simulink library "rov_design_analysis"  (Simulink 6.0)
settings: Solver=ode45  SolverMode=SingleTasking  StartTime=0.0  StopTime=10.0  RelTol=1e-3
undefined symbols (not defined in the file or in its folder): amp, At, B, Bt, Ct, cycles, D, den, DL, Do, DQ, DQL, freq, frtest, I, L, m, M, Ma, magnitude, MaU, Mt, nmiss, num, phase, rg, sigbuilder_block, slcm, T, W, xb, xg, Xudot, yb, yg, Yvdot, zb, zg, Zwdot
libraries: simulink_extras x32, simulink x27, rov_design_analysis x15, marine_gnc x10, dspmtrx2 x6, dspstat3 x4
(part 6 of 9)

== system rov_design_analysis/ROV Controller /Hybrid Control- one DoF/Body-fixed to Earth_fixed Transformation1/Transformation matrix T ==
  translational body velocity : Inport  Port=1  LatchInput=off
  angular position : Inport  Port=2  LatchInput=off
  Mux : Mux  Inputs=3
  Row1 of R : Subsystem
      mask Display: disp('Row 1')
  Row2 of R : Subsystem
      mask Display: disp('Row 2')
  Row3 of R : Subsystem
      mask Display: disp('Row 3')
  translational earth velocity : Outport  InitialOutput=0
  wires:
  Mux/1 -> translational earth velocity/1
  Row3 of R/1(translational earth velocity (row 3)) -> Mux/3
  Row2 of R/1(translational earth velocity (row 2)) -> Mux/2
  Row1 of R/1(translational earth velocity (row 1)) -> Mux/1
  angular position/1 -> Row3 of R/2(angular position), Row1 of R/2(angular position), Row2 of R/2(angular position)
  translational body velocity/1 -> Row1 of R/1(translational body velocity), Row2 of R/1(translational body velocity), Row3 of R/1(translational body velocity)

== system rov_design_analysis/ROV Controller /Hybrid Control- one DoF/Body-fixed to Earth_fixed Transformation3/Transformation matrix R ==
  angular body  velocity : Inport  Port=1  LatchInput=off
  angular position : Inport  Port=2  LatchInput=off
  Mux : Mux  Inputs=3
  Row1 of T : Subsystem
      mask Display: disp('Row 1')
  Row2 of T : Subsystem
      mask Display: disp('Row 2')
  Row3 of T : Subsystem
      mask Display: disp('Row 3')
  angular earth velocity : Outport  InitialOutput=0
  wires:
  angular body  velocity/1 -> Row1 of T/1(angular body  velocity), Row2 of T/1("angular body velocity "), Row3 of T/1("angular body velocity ")
  Row1 of T/1(angular earth velocity (row 1)) -> Mux/1
  Row2 of T/1(angular earth velocity (row 2)) -> Mux/2
  Row3 of T/1(angular earth velocity (row 3)) -> Mux/3
  Mux/1 -> angular earth velocity/1
  angular position/1 -> Row2 of T/2(angular position), Row1 of T/2(angular position), Row3 of T/2(angular position)

== system rov_design_analysis/ROV Controller /Hybrid Control- one DoF/Body-fixed to Earth_fixed Transformation3/Transformation matrix T ==
  translational body velocity : Inport  Port=1  LatchInput=off
  angular position : Inport  Port=2  LatchInput=off
  Mux : Mux  Inputs=3
  Row1 of R : Subsystem
      mask Display: disp('Row 1')
  Row2 of R : Subsystem
      mask Display: disp('Row 2')
  Row3 of R : Subsystem
      mask Display: disp('Row 3')
  translational earth velocity : Outport  InitialOutput=0
  wires:
  translational body velocity/1 -> Row3 of R/1(translational body velocity), Row2 of R/1(translational body velocity), Row1 of R/1(translational body velocity)
  angular position/1 -> Row2 of R/2(angular position), Row1 of R/2(angular position), Row3 of R/2(angular position)
  Row1 of R/1(translational earth velocity (row 1)) -> Mux/1
  Row2 of R/1(translational earth velocity (row 2)) -> Mux/2
  Row3 of R/1(translational earth velocity (row 3)) -> Mux/3
  Mux/1 -> translational earth velocity/1

== system rov_design_analysis/ROV Controller /Hybrid Control- one DoF/Subsystem2/SubSystem11 ==
  volt : Inport  Port=1  LatchInput=off
  Transfer Fcn : TransferFcn  Numerator=[3700 0.037]  Denominator=[0.5 847.5 76000]
  thrust : Outport
  wires:
  Transfer Fcn/1 -> thrust/1
  volt/1 -> Transfer Fcn/1

== system rov_design_analysis/ROV Controller /Hybrid Control- one DoF/Subsystem2/SubSystem12 ==
  volt : Inport  Port=1  LatchInput=off
  Transfer Fcn : TransferFcn  Numerator=[3700 0.037]  Denominator=[0.5 847.5 76000]
  thrust : Outport
  wires:
  Transfer Fcn/1 -> thrust/1
  volt/1 -> Transfer Fcn/1

== system rov_design_analysis/ROV Controller /Hybrid Control- one DoF/Subsystem2/SubSystem5 ==
  volt : Inport  Port=1  LatchInput=off
  Transfer Fcn : TransferFcn  Numerator=[3700 0.037]  Denominator=[0.5 847.5 76000]
  thrust : Outport
  wires:
  Transfer Fcn/1 -> thrust/1
  volt/1 -> Transfer Fcn/1

== system rov_design_analysis/ROV Controller /Hybrid Control- one DoF/Subsystem2/SubSystem6 ==
  volt : Inport  Port=1  LatchInput=off
  Transfer Fcn : TransferFcn  Numerator=[3700 0.037]  Denominator=[0.5 847.5 76000]
  thrust : Outport
  wires:
  Transfer Fcn/1 -> thrust/1
  volt/1 -> Transfer Fcn/1

== system rov_design_analysis/ROV Controller /Nonlinear-Based PD  Cascaded  Controller - 6 DoF/Body-fixed to Earth_fixed Transformation1/Transformation matrix R ==
  angular body  velocity : Inport  Port=1  LatchInput=off
  angular position : Inport  Port=2  LatchInput=off
  Mux : Mux  Inputs=3
  Row1 of T : Subsystem
      mask Display: disp('Row 1')
  Row2 of T : Subsystem
      mask Display: disp('Row 2')
  Row3 of T : Subsystem
      mask Display: disp('Row 3')
  angular earth velocity : Outport  InitialOutput=0
  wires:
  angular position/1 -> Row3 of T/2(angular position), Row1 of T/2(angular position), Row2 of T/2(angular position)
  Mux/1 -> angular earth velocity/1
  Row3 of T/1(angular earth velocity (row 3)) -> Mux/3
  Row2 of T/1(angular earth velocity (row 2)) -> Mux/2
  Row1 of T/1(angular earth velocity (row 1)) -> Mux/1
  angular body  velocity/1 -> Row3 of T/1("angular body velocity "), Row2 of T/1("angular body velocity "), Row1 of T/1(angular body  velocity)

== system rov_design_analysis/ROV Controller /Nonlinear-Based PD  Cascaded  Controller - 6 DoF/Body-fixed to Earth_fixed Transformation1/Transformation matrix T ==
  translational body velocity : Inport  Port=1  LatchInput=off
  angular position : Inport  Port=2  LatchInput=off
  Mux : Mux  Inputs=3
  Row1 of R : Subsystem
      mask Display: disp('Row 1')
  Row2 of R : Subsystem
      mask Display: disp('Row 2')
  Row3 of R : Subsystem
      mask Display: disp('Row 3')
  translational earth velocity : Outport  InitialOutput=0
  wires:
  Mux/1 -> translational earth velocity/1
  Row3 of R/1(translational earth velocity (row 3)) -> Mux/3
  Row2 of R/1(translational earth velocity (row 2)) -> Mux/2
  Row1 of R/1(translational earth velocity (row 1)) -> Mux/1
  angular position/1 -> Row3 of R/2(angular position), Row1 of R/2(angular position), Row2 of R/2(angular position)
  translational body velocity/1 -> Row1 of R/1(translational body velocity), Row2 of R/1(translational body velocity), Row3 of R/1(translational body velocity)

== system rov_design_analysis/ROV Controller /Nonlinear-Based PD  Cascaded  Controller - 6 DoF/Body-fixed to Earth_fixed Transformation3/Transformation matrix R ==
  angular body  velocity : Inport  Port=1  LatchInput=off
  angular position : Inport  Port=2  LatchInput=off
  Mux : Mux  Inputs=3
  Row1 of T : Subsystem
      mask Display: disp('Row 1')
  Row2 of T : Subsystem
      mask Display: disp('Row 2')
  Row3 of T : Subsystem
      mask Display: disp('Row 3')
  angular earth velocity : Outport  InitialOutput=0
  wires:
  angular body  velocity/1 -> Row1 of T/1(angular body  velocity), Row2 of T/1("angular body velocity "), Row3 of T/1("angular body velocity ")
  Row1 of T/1(angular earth velocity (row 1)) -> Mux/1
  Row2 of T/1(angular earth velocity (row 2)) -> Mux/2
  Row3 of T/1(angular earth velocity (row 3)) -> Mux/3
  Mux/1 -> angular earth velocity/1
  angular position/1 -> Row2 of T/2(angular position), Row1 of T/2(angular position), Row3 of T/2(angular position)

== system rov_design_analysis/ROV Controller /Nonlinear-Based PD  Cascaded  Controller - 6 DoF/Body-fixed to Earth_fixed Transformation3/Transformation matrix T ==
  translational body velocity : Inport  Port=1  LatchInput=off
  angular position : Inport  Port=2  LatchInput=off
  Mux : Mux  Inputs=3
  Row1 of R : Subsystem
      mask Display: disp('Row 1')
  Row2 of R : Subsystem
      mask Display: disp('Row 2')
  Row3 of R : Subsystem
      mask Display: disp('Row 3')
  translational earth velocity : Outport  InitialOutput=0
  wires:
  translational body velocity/1 -> Row3 of R/1(translational body velocity), Row2 of R/1(translational body velocity), Row1 of R/1(translational body velocity)
  angular position/1 -> Row2 of R/2(angular position), Row1 of R/2(angular position), Row3 of R/2(angular position)
  Row1 of R/1(translational earth velocity (row 1)) -> Mux/1
  Row2 of R/1(translational earth velocity (row 2)) -> Mux/2
  Row3 of R/1(translational earth velocity (row 3)) -> Mux/3
  Mux/1 -> translational earth velocity/1

== system rov_design_analysis/ROV Controller /Nonlinear-Based PD  Cascaded  Controller - 6 DoF/Subsystem2/SubSystem11 ==
  volt : Inport  Port=1  LatchInput=off
  Transfer Fcn : TransferFcn  Numerator=[3700 0.037]  Denominator=[0.5 847.5 76000]
  thrust : Outport
  wires:
  Transfer Fcn/1 -> thrust/1
  volt/1 -> Transfer Fcn/1

== system rov_design_analysis/ROV Controller /Nonlinear-Based PD  Cascaded  Controller - 6 DoF/Subsystem2/SubSystem12 ==
  volt : Inport  Port=1  LatchInput=off
  Transfer Fcn : TransferFcn  Numerator=[3700 0.037]  Denominator=[0.5 847.5 76000]
  thrust : Outport
  wires:
  Transfer Fcn/1 -> thrust/1
  volt/1 -> Transfer Fcn/1

== system rov_design_analysis/ROV Controller /Nonlinear-Based PD  Cascaded  Controller - 6 DoF/Subsystem2/SubSystem5 ==
  volt : Inport  Port=1  LatchInput=off
  Transfer Fcn : TransferFcn  Numerator=[3700 0.037]  Denominator=[0.5 847.5 76000]
  thrust : Outport
  wires:
  Transfer Fcn/1 -> thrust/1
  volt/1 -> Transfer Fcn/1

== system rov_design_analysis/ROV Controller /Nonlinear-Based PD  Cascaded  Controller - 6 DoF/Subsystem2/SubSystem6 ==
  volt : Inport  Port=1  LatchInput=off
  Transfer Fcn : TransferFcn  Numerator=[3700 0.037]  Denominator=[0.5 847.5 76000]
  thrust : Outport
  wires:
  Transfer Fcn/1 -> thrust/1
  volt/1 -> Transfer Fcn/1

== system rov_design_analysis/ROV Controller /Nonlinear-Sliding-Mode Cascaded  Controller - 6 DoF/Body-fixed to Earth_fixed Transformation1/Transformation matrix R ==
  angular body  velocity : Inport  Port=1  LatchInput=off
  angular position : Inport  Port=2  LatchInput=off
  Mux : Mux  Inputs=3
  Row1 of T : Subsystem
      mask Display: disp('Row 1')
  Row2 of T : Subsystem
      mask Display: disp('Row 2')
  Row3 of T : Subsystem
      mask Display: disp('Row 3')
  angular earth velocity : Outport  InitialOutput=0
  wires:
  angular body  velocity/1 -> Row1 of T/1(angular body  velocity), Row2 of T/1("angular body velocity "), Row3 of T/1("angular body velocity ")
  Row1 of T/1(angular earth velocity (row 1)) -> Mux/1
  Row2 of T/1(angular earth velocity (row 2)) -> Mux/2
  Row3 of T/1(angular earth velocity (row 3)) -> Mux/3
  Mux/1 -> angular earth velocity/1
  angular position/1 -> Row2 of T/2(angular position), Row1 of T/2(angular position), Row3 of T/2(angular position)

== system rov_design_analysis/ROV Controller /Nonlinear-Sliding-Mode Cascaded  Controller - 6 DoF/Body-fixed to Earth_fixed Transformation1/Transformation matrix T ==
  translational body velocity : Inport  Port=1  LatchInput=off
  angular position : Inport  Port=2  LatchInput=off
  Mux : Mux  Inputs=3
  Row1 of R : Subsystem
      mask Display: disp('Row 1')
  Row2 of R : Subsystem
      mask Display: disp('Row 2')
  Row3 of R : Subsystem
      mask Display: disp('Row 3')
  translational earth velocity : Outport  InitialOutput=0
  wires:
  translational body velocity/1 -> Row3 of R/1(translational body velocity), Row2 of R/1(translational body velocity), Row1 of R/1(translational body velocity)
  angular position/1 -> Row2 of R/2(angular position), Row1 of R/2(angular position), Row3 of R/2(angular position)
  Row1 of R/1(translational earth velocity (row 1)) -> Mux/1
  Row2 of R/1(translational earth velocity (row 2)) -> Mux/2
  Row3 of R/1(translational earth velocity (row 3)) -> Mux/3
  Mux/1 -> translational earth velocity/1

== system rov_design_analysis/ROV Controller /Nonlinear-Sliding-Mode Cascaded  Controller - 6 DoF/Body-fixed to Earth_fixed Transformation3/Transformation matrix R ==
  angular body  velocity : Inport  Port=1  LatchInput=off
  angular position : Inport  Port=2  LatchInput=off
  Mux : Mux  Inputs=3
  Row1 of T : Subsystem
      mask Display: disp('Row 1')
  Row2 of T : Subsystem
      mask Display: disp('Row 2')
  Row3 of T : Subsystem
      mask Display: disp('Row 3')
  angular earth velocity : Outport  InitialOutput=0
  wires:
  angular position/1 -> Row3 of T/2(angular position), Row1 of T/2(angular position), Row2 of T/2(angular position)
  Mux/1 -> angular earth velocity/1
  Row3 of T/1(angular earth velocity (row 3)) -> Mux/3
  Row2 of T/1(angular earth velocity (row 2)) -> Mux/2
  Row1 of T/1(angular earth velocity (row 1)) -> Mux/1
  angular body  velocity/1 -> Row3 of T/1("angular body velocity "), Row2 of T/1("angular body velocity "), Row1 of T/1(angular body  velocity)

== system rov_design_analysis/ROV Controller /Nonlinear-Sliding-Mode Cascaded  Controller - 6 DoF/Body-fixed to Earth_fixed Transformation3/Transformation matrix T ==
  translational body velocity : Inport  Port=1  LatchInput=off
  angular position : Inport  Port=2  LatchInput=off
  Mux : Mux  Inputs=3
  Row1 of R : Subsystem
      mask Display: disp('Row 1')
  Row2 of R : Subsystem
      mask Display: disp('Row 2')
  Row3 of R : Subsystem
      mask Display: disp('Row 3')
  translational earth velocity : Outport  InitialOutput=0
  wires:
  Mux/1 -> translational earth velocity/1
  Row3 of R/1(translational earth velocity (row 3)) -> Mux/3
  Row2 of R/1(translational earth velocity (row 2)) -> Mux/2
  Row1 of R/1(translational earth velocity (row 1)) -> Mux/1
  angular position/1 -> Row3 of R/2(angular position), Row1 of R/2(angular position), Row2 of R/2(angular position)
  translational body velocity/1 -> Row1 of R/1(translational body velocity), Row2 of R/1(translational body velocity), Row3 of R/1(translational body velocity)

== system rov_design_analysis/ROV Controller /Nonlinear-Sliding-Mode Cascaded  Controller - 6 DoF/Subsystem2/SubSystem11 ==
  volt : Inport  Port=1  LatchInput=off
  Transfer Fcn : TransferFcn  Numerator=[3700 0.037]  Denominator=[0.5 847.5 76000]
  thrust : Outport
  wires:
  volt/1 -> Transfer Fcn/1
  Transfer Fcn/1 -> thrust/1

== system rov_design_analysis/ROV Controller /Nonlinear-Sliding-Mode Cascaded  Controller - 6 DoF/Subsystem2/SubSystem12 ==
  volt : Inport  Port=1  LatchInput=off
  Transfer Fcn : TransferFcn  Numerator=[3700 0.037]  Denominator=[0.5 847.5 76000]
  thrust : Outport
  wires:
  volt/1 -> Transfer Fcn/1
  Transfer Fcn/1 -> thrust/1

== system rov_design_analysis/ROV Controller /Nonlinear-Sliding-Mode Cascaded  Controller - 6 DoF/Subsystem2/SubSystem5 ==
  volt : Inport  Port=1  LatchInput=off
  Transfer Fcn : TransferFcn  Numerator=[3700 0.037]  Denominator=[0.5 847.5 76000]
  thrust : Outport
  wires:
  volt/1 -> Transfer Fcn/1
  Transfer Fcn/1 -> thrust/1

== system rov_design_analysis/ROV Controller /Nonlinear-Sliding-Mode Cascaded  Controller - 6 DoF/Subsystem2/SubSystem6 ==
  volt : Inport  Port=1  LatchInput=off
  Transfer Fcn : TransferFcn  Numerator=[3700 0.037]  Denominator=[0.5 847.5 76000]
  thrust : Outport
  wires:
  volt/1 -> Transfer Fcn/1
  Transfer Fcn/1 -> thrust/1

== system rov_design_analysis/ROV Controller /P-Decoupled  Cascaded loop Controller  - 6 DoF/Body-fixed to Earth_fixed Transformation1/Transformation matrix R ==
  angular body  velocity : Inport  Port=1  LatchInput=off
  angular position : Inport  Port=2  LatchInput=off
  Mux : Mux  Inputs=3
  Row1 of T : Subsystem
      mask Display: disp('Row 1')
  Row2 of T : Subsystem
      mask Display: disp('Row 2')
  Row3 of T : Subsystem
      mask Display: disp('Row 3')
  angular earth velocity : Outport  InitialOutput=0
  wires:
  angular body  velocity/1 -> Row1 of T/1(angular body  velocity), Row2 of T/1("angular body velocity "), Row3 of T/1("angular body velocity ")
  Row1 of T/1(angular earth velocity (row 1)) -> Mux/1
  Row2 of T/1(angular earth velocity (row 2)) -> Mux/2
  Row3 of T/1(angular earth velocity (row 3)) -> Mux/3
  Mux/1 -> angular earth velocity/1
  angular position/1 -> Row2 of T/2(angular position), Row1 of T/2(angular position), Row3 of T/2(angular position)

== system rov_design_analysis/ROV Controller /P-Decoupled  Cascaded loop Controller  - 6 DoF/Body-fixed to Earth_fixed Transformation1/Transformation matrix T ==
  translational body velocity : Inport  Port=1  LatchInput=off
  angular position : Inport  Port=2  LatchInput=off
  Mux : Mux  Inputs=3
  Row1 of R : Subsystem
      mask Display: disp('Row 1')
  Row2 of R : Subsystem
      mask Display: disp('Row 2')
  Row3 of R : Subsystem
      mask Display: disp('Row 3')
  translational earth velocity : Outport  InitialOutput=0
  wires:
  translational body velocity/1 -> Row3 of R/1(translational body velocity), Row2 of R/1(translational body velocity), Row1 of R/1(translational body velocity)
  angular position/1 -> Row2 of R/2(angular position), Row1 of R/2(angular position), Row3 of R/2(angular position)
  Row1 of R/1(translational earth velocity (row 1)) -> Mux/1
  Row2 of R/1(translational earth velocity (row 2)) -> Mux/2
  Row3 of R/1(translational earth velocity (row 3)) -> Mux/3
  Mux/1 -> translational earth velocity/1

== system rov_design_analysis/ROV Controller /P-Decoupled  Cascaded loop Controller  - 6 DoF/Body-fixed to Earth_fixed Transformation3/Transformation matrix R ==
  angular body  velocity : Inport  Port=1  LatchInput=off
  angular position : Inport  Port=2  LatchInput=off
  Mux : Mux  Inputs=3
  Row1 of T : Subsystem
      mask Display: disp('Row 1')
  Row2 of T : Subsystem
      mask Display: disp('Row 2')
  Row3 of T : Subsystem
      mask Display: disp('Row 3')
  angular earth velocity : Outport  InitialOutput=0
  wires:
  angular position/1 -> Row3 of T/2(angular position), Row1 of T/2(angular position), Row2 of T/2(angular position)
  Mux/1 -> angular earth velocity/1
  Row3 of T/1(angular earth velocity (row 3)) -> Mux/3
  Row2 of T/1(angular earth velocity (row 2)) -> Mux/2
  Row1 of T/1(angular earth velocity (row 1)) -> Mux/1
  angular body  velocity/1 -> Row3 of T/1("angular body velocity "), Row2 of T/1("angular body velocity "), Row1 of T/1(angular body  velocity)

== system rov_design_analysis/ROV Controller /P-Decoupled  Cascaded loop Controller  - 6 DoF/Body-fixed to Earth_fixed Transformation3/Transformation matrix T ==
  translational body velocity : Inport  Port=1  LatchInput=off
  angular position : Inport  Port=2  LatchInput=off
  Mux : Mux  Inputs=3
  Row1 of R : Subsystem
      mask Display: disp('Row 1')
  Row2 of R : Subsystem
      mask Display: disp('Row 2')
  Row3 of R : Subsystem
      mask Display: disp('Row 3')
  translational earth velocity : Outport  InitialOutput=0
  wires:
  Mux/1 -> translational earth velocity/1
  Row3 of R/1(translational earth velocity (row 3)) -> Mux/3
  Row2 of R/1(translational earth velocity (row 2)) -> Mux/2
  Row1 of R/1(translational earth velocity (row 1)) -> Mux/1
  angular position/1 -> Row3 of R/2(angular position), Row1 of R/2(angular position), Row2 of R/2(angular position)
  translational body velocity/1 -> Row1 of R/1(translational body velocity), Row2 of R/1(translational body velocity), Row3 of R/1(translational body velocity)

== system rov_design_analysis/ROV Controller /P-Decoupled  Cascaded loop Controller  - 6 DoF/Subsystem2/SubSystem11 ==
  volt : Inport  Port=1  LatchInput=off
  Transfer Fcn : TransferFcn  Numerator=[3700 0.037]  Denominator=[0.5 847.5 76000]
  thrust : Outport
  wires:
  volt/1 -> Transfer Fcn/1
  Transfer Fcn/1 -> thrust/1

== system rov_design_analysis/ROV Controller /P-Decoupled  Cascaded loop Controller  - 6 DoF/Subsystem2/SubSystem12 ==
  volt : Inport  Port=1  LatchInput=off
  Transfer Fcn : TransferFcn  Numerator=[3700 0.037]  Denominator=[0.5 847.5 76000]
  thrust : Outport
  wires:
  volt/1 -> Transfer Fcn/1
  Transfer Fcn/1 -> thrust/1

== system rov_design_analysis/ROV Controller /P-Decoupled  Cascaded loop Controller  - 6 DoF/Subsystem2/SubSystem5 ==
  volt : Inport  Port=1  LatchInput=off
  Transfer Fcn : TransferFcn  Numerator=[3700 0.037]  Denominator=[0.5 847.5 76000]
  thrust : Outport
  wires:
  volt/1 -> Transfer Fcn/1
  Transfer Fcn/1 -> thrust/1

== system rov_design_analysis/ROV Controller /P-Decoupled  Cascaded loop Controller  - 6 DoF/Subsystem2/SubSystem6 ==
  volt : Inport  Port=1  LatchInput=off
  Transfer Fcn : TransferFcn  Numerator=[3700 0.037]  Denominator=[0.5 847.5 76000]
  thrust : Outport
  wires:
  volt/1 -> Transfer Fcn/1
  Transfer Fcn/1 -> thrust/1

== system rov_design_analysis/ROV Controller /P-Decoupled  Single loop Controller - 6 DoF /Body-fixed to Earth_fixed Transformation1/Transformation matrix R ==
  angular body  velocity : Inport  Port=1  LatchInput=off
  angular position : Inport  Port=2  LatchInput=off
  Mux : Mux  Inputs=3
  Row1 of T : Subsystem
      mask Display: disp('Row 1')
  Row2 of T : Subsystem
      mask Display: disp('Row 2')
  Row3 of T : Subsystem
      mask Display: disp('Row 3')
  angular earth velocity : Outport  InitialOutput=0
  wires:
  angular position/1 -> Row3 of T/2(angular position), Row1 of T/2(angular position), Row2 of T/2(angular position)
  Mux/1 -> angular earth velocity/1
  Row3 of T/1(angular earth velocity (row 3)) -> Mux/3
  Row2 of T/1(angular earth velocity (row 2)) -> Mux/2
  Row1 of T/1(angular earth velocity (row 1)) -> Mux/1
  angular body  velocity/1 -> Row3 of T/1("angular body velocity "), Row2 of T/1("angular body velocity "), Row1 of T/1(angular body  velocity)

== system rov_design_analysis/ROV Controller /P-Decoupled  Single loop Controller - 6 DoF /Body-fixed to Earth_fixed Transformation1/Transformation matrix T ==
  translational body velocity : Inport  Port=1  LatchInput=off
  angular position : Inport  Port=2  LatchInput=off
  Mux : Mux  Inputs=3
  Row1 of R : Subsystem
      mask Display: disp('Row 1')
  Row2 of R : Subsystem
      mask Display: disp('Row 2')
  Row3 of R : Subsystem
      mask Display: disp('Row 3')
  translational earth velocity : Outport  InitialOutput=0
  wires:
  Mux/1 -> translational earth velocity/1
  Row3 of R/1(translational earth velocity (row 3)) -> Mux/3
  Row2 of R/1(translational earth velocity (row 2)) -> Mux/2
  Row1 of R/1(translational earth velocity (row 1)) -> Mux/1
  angular position/1 -> Row3 of R/2(angular position), Row1 of R/2(angular position), Row2 of R/2(angular position)
  translational body velocity/1 -> Row1 of R/1(translational body velocity), Row2 of R/1(translational body velocity), Row3 of R/1(translational body velocity)

== system rov_design_analysis/ROV Controller /P-Decoupled  Single loop Controller - 6 DoF /Body-fixed to Earth_fixed Transformation3/Transformation matrix R ==
  angular body  velocity : Inport  Port=1  LatchInput=off
  angular position : Inport  Port=2  LatchInput=off
  Mux : Mux  Inputs=3
  Row1 of T : Subsystem
      mask Display: disp('Row 1')
  Row2 of T : Subsystem
      mask Display: disp('Row 2')
  Row3 of T : Subsystem
      mask Display: disp('Row 3')
  angular earth velocity : Outport  InitialOutput=0
  wires:
  angular body  velocity/1 -> Row1 of T/1(angular body  velocity), Row2 of T/1("angular body velocity "), Row3 of T/1("angular body velocity ")
  Row1 of T/1(angular earth velocity (row 1)) -> Mux/1
  Row2 of T/1(angular earth velocity (row 2)) -> Mux/2
  Row3 of T/1(angular earth velocity (row 3)) -> Mux/3
  Mux/1 -> angular earth velocity/1
  angular position/1 -> Row2 of T/2(angular position), Row1 of T/2(angular position), Row3 of T/2(angular position)

== system rov_design_analysis/ROV Controller /P-Decoupled  Single loop Controller - 6 DoF /Body-fixed to Earth_fixed Transformation3/Transformation matrix T ==
  translational body velocity : Inport  Port=1  LatchInput=off
  angular position : Inport  Port=2  LatchInput=off
  Mux : Mux  Inputs=3
  Row1 of R : Subsystem
      mask Display: disp('Row 1')
  Row2 of R : Subsystem
      mask Display: disp('Row 2')
  Row3 of R : Subsystem
      mask Display: disp('Row 3')
  translational earth velocity : Outport  InitialOutput=0
  wires:
  translational body velocity/1 -> Row3 of R/1(translational body velocity), Row2 of R/1(translational body velocity), Row1 of R/1(translational body velocity)
  angular position/1 -> Row2 of R/2(angular position), Row1 of R/2(angular position), Row3 of R/2(angular position)
  Row1 of R/1(translational earth velocity (row 1)) -> Mux/1
  Row2 of R/1(translational earth velocity (row 2)) -> Mux/2
  Row3 of R/1(translational earth velocity (row 3)) -> Mux/3
  Mux/1 -> translational earth velocity/1

== system rov_design_analysis/ROV Controller /P-Decoupled  Single loop Controller - 6 DoF /Subsystem2/SubSystem11 ==
  volt : Inport  Port=1  LatchInput=off
  Transfer Fcn : TransferFcn  Numerator=[3700 0.037]  Denominator=[0.5 847.5 76000]
  thrust : Outport
  wires:
  Transfer Fcn/1 -> thrust/1
  volt/1 -> Transfer Fcn/1

== system rov_design_analysis/ROV Controller /P-Decoupled  Single loop Controller - 6 DoF /Subsystem2/SubSystem12 ==
  volt : Inport  Port=1  LatchInput=off
  Transfer Fcn : TransferFcn  Numerator=[3700 0.037]  Denominator=[0.5 847.5 76000]
  thrust : Outport
  wires:
  Transfer Fcn/1 -> thrust/1
  volt/1 -> Transfer Fcn/1

== system rov_design_analysis/ROV Controller /P-Decoupled  Single loop Controller - 6 DoF /Subsystem2/SubSystem5 ==
  volt : Inport  Port=1  LatchInput=off
  Transfer Fcn : TransferFcn  Numerator=[3700 0.037]  Denominator=[0.5 847.5 76000]
  thrust : Outport
  wires:
  Transfer Fcn/1 -> thrust/1
  volt/1 -> Transfer Fcn/1

== system rov_design_analysis/ROV Controller /P-Decoupled  Single loop Controller - 6 DoF /Subsystem2/SubSystem6 ==
  volt : Inport  Port=1  LatchInput=off
  Transfer Fcn : TransferFcn  Numerator=[3700 0.037]  Denominator=[0.5 847.5 76000]
  thrust : Outport
  wires:
  Transfer Fcn/1 -> thrust/1
  volt/1 -> Transfer Fcn/1

== system rov_design_analysis/ROV Controller /ROV design  in earth fixed frame  PID - 6 DoF/Model Info/EmptySubsystem ==

== system rov_design_analysis/Thruster  Controller/1. Propeller thrust control - one DoF/Speed control/Shaft Dynamic ==
  Qm : Inport  Port=1  LatchInput=off
  Qa : Inport  Port=2  LatchInput=off
  2*pi : Constant  Value=2*pi
  Integrator : Integrator
  Km : Gain  Orientation=left  Gain=12.562  SaturateOnIntegerOverflow=on
  Math Function : Math  Operator=reciprocal  SaturateOnIntegerOverflow=on
  Product : Product  Inputs=3  SaturateOnIntegerOverflow=on  RndMeth=Zero  InputSameDT=on
  Sum : Sum  Inputs=|+--  SaturateOnIntegerOverflow=on  InputSameDT=on
  shaft inertia : Constant  Value=0.0492
  n : Outport
  wires:
  2*pi/1 -> Product/1
  Math Function/1 -> Product/2
  shaft inertia/1 -> Math Function/1
  Product/1 -> Integrator/1
  Sum/1 -> Product/3
  Km/1 -> Sum/3
  Integrator/1 -> n/1, Km/1
  Qm/1 -> Sum/1
  Qa/1 -> Sum/2

== system rov_design_analysis/Thruster  Controller/1. Propeller thrust control - one DoF/Speed control/first order motor dynamic ==
  Qc : Inport  Port=1  LatchInput=off
  1/time const : Constant  Value=0.1
  Integrator : Integrator
  Product : Product  SaturateOnIntegerOverflow=on  RndMeth=Zero  InputSameDT=on
  Sum : Sum  Inputs=|+-  SaturateOnIntegerOverflow=on  InputSameDT=on
  Qm : Outport
  wires:
  1/time const/1 -> Product/1
  Product/1 -> Sum/1
  Sum/1 -> Integrator/1
  Integrator/1 -> Sum/2, Qm/1
  Qc/1 -> Product/2

== system rov_design_analysis/Thruster  Controller/1. Propeller thrust control - one DoF/Speed control/propeller Load Torque ==
  n : Inport  Port=1  LatchInput=off
  Abs : Abs  Orientation=left  SaturateOnIntegerOverflow=on
  Constant4 : Constant  Orientation=left  Value=5
  D : Constant  Orientation=left  Value=0.1
  KQ : Constant  Orientation=left  Value=0.000272
  Math Function1 : Math  Orientation=left  Operator=pow  SaturateOnIntegerOverflow=on
  Product1 : Product  Orientation=left  Inputs=5  SaturateOnIntegerOverflow=on  RndMeth=Zero  InputSameDT=on
  "seawater density " : Constant  Orientation=left  Value=1024
  Qa : Outport
  wires:
  "seawater density "/1 -> Product1/1
  Math Function1/1 -> Product1/2
  KQ/1 -> Product1/3
  Abs/1 -> Product1/4
  n/1 -> Abs/1, Product1/5
  Product1/1 -> Qa/1
  D/1 -> Math Function1/1
  Constant4/1 -> Math Function1/2

== system rov_design_analysis/Thruster  Controller/1. Propeller thrust control - one DoF/Speed control/propeller thruster ==
  n : Inport  Port=1  LatchInput=off
  Abs : Abs  Orientation=left  SaturateOnIntegerOverflow=on
  Constant4 : Constant  Orientation=left  Value=4
  D : Constant  Orientation=left  Value=0.1
  KT : Constant  Orientation=left  Value=0.0027
  Math Function1 : Math  Orientation=left  Operator=pow  SaturateOnIntegerOverflow=on
  Product1 : Product  Orientation=left  Inputs=5  SaturateOnIntegerOverflow=on  RndMeth=Zero  InputSameDT=on
  pw : Constant  Orientation=left  Value=1024
  Ta : Outport
  wires:
  pw/1 -> Product1/1
  Math Function1/1 -> Product1/2
  KT/1 -> Product1/3
  Abs/1 -> Product1/4
  n/1 -> Abs/1, Product1/5
  Product1/1 -> Ta/1
  D/1 -> Math Function1/1
  Constant4/1 -> Math Function1/2

== system rov_design_analysis/Thruster  Controller/1. Propeller thrust control - one DoF/Speed control/propeller thruster       ==
  Tref : Inport  Port=1  LatchInput=off
  Abs : Abs  Orientation=left  SaturateOnIntegerOverflow=on
  Constant4 : Constant  Orientation=left  Value=4
  D : Constant  Orientation=left  Value=0.1
  KTo : Constant  Orientation=left  Value=0.0027
  Math Function1 : Math  Orientation=left  Operator=pow  SaturateOnIntegerOverflow=on
  Math Function2 : Math  Orientation=left  Operator=reciprocal  SaturateOnIntegerOverflow=on
  Math Function3 : Math  Orientation=left  Operator=sqrt  SaturateOnIntegerOverflow=on
  Product1 : Product  Orientation=left  Inputs=3  SaturateOnIntegerOverflow=on  RndMeth=Zero  InputSameDT=on
  Product2 : Product  Orientation=left  SaturateOnIntegerOverflow=on  RndMeth=Zero  InputSameDT=on
  Product3 : Product  Orientation=left  SaturateOnIntegerOverflow=on  RndMeth=Zero  InputSameDT=on
  Sign : Signum  Orientation=left
  pw : Constant  Orientation=left  Value=1024
  nref : Outport
  wires:
  pw/1 -> Product1/1
  Math Function1/1 -> Product1/2
  KTo/1 -> Product1/3
  Product1/1 -> Math Function2/1
  Math Function2/1 -> Product2/1
  Product2/1 -> Abs/1
  Abs/1 -> Math Function3/1
  Math Function3/1 -> Product3/2
  Product3/1 -> nref/1
  Sign/1 -> Product3/1
  Tref/1 -> Sign/1, Product2/2
  D/1 -> Math Function1/1
  Constant4/1 -> Math Function1/2

== system rov_design_analysis/Thruster  Controller/2. Thruster Allocation- RRC ROV/thruster allocation /Atomic Subsystem1 ==
  In2 : Inport  Port=1  LatchInput=off
  Abs : Abs
  Product1 : Product  OutDataTypeMode=double  SaturateOnIntegerOverflow=on  RndMeth=Zero
  Product5 : Product  OutDataTypeMode=double  SaturateOnIntegerOverflow=on  RndMeth=Zero
  Sign1 : Signum
  Switch1 : Switch  Threshold=1  SaturateOnIntegerOverflow=on  InputSameDT=on
  <0 : Outport
  wires:
  Sign1/1 -> Product1/2, Product5/1, Switch1/2
  Product1/1 -> Switch1/1
  Product5/1 -> Switch1/3
  Switch1/1 -> <0/1
  In2/1 -> Sign1/1, Product1/1, Abs/1
  Abs/1 -> Product5/2

== system rov_design_analysis/Thruster  Controller/2. Thruster Allocation- RRC ROV/thruster allocation /Atomic Subsystem2 ==
  In2 : Inport  Port=1  LatchInput=off
  Abs : Abs
  Product1 : Product  OutDataTypeMode=double  SaturateOnIntegerOverflow=on  RndMeth=Zero
  Product5 : Product  OutDataTypeMode=double  SaturateOnIntegerOverflow=on  RndMeth=Zero
  Sign1 : Signum
  Switch1 : Switch  Threshold=1  SaturateOnIntegerOverflow=on  InputSameDT=on
  <0 : Outport
  wires:
  In2/1 -> Sign1/1, Product1/1, Abs/1
  Sign1/1 -> Switch1/2, Product1/2, Product5/1
  Product1/1 -> Switch1/1
  Product5/1 -> Switch1/3
  Switch1/1 -> <0/1
  Abs/1 -> Product5/2

== system rov_design_analysis/Thruster  Controller/2. Thruster Allocation- RRC ROV/thruster allocation /Atomic Subsystem3 ==
  In2 : Inport  Port=1  LatchInput=off
  Abs : Abs
  Product1 : Product  OutDataTypeMode=double  SaturateOnIntegerOverflow=on  RndMeth=Zero
  Product5 : Product  OutDataTypeMode=double  SaturateOnIntegerOverflow=on  RndMeth=Zero
  Sign1 : Signum
  Switch1 : Switch  Threshold=1  SaturateOnIntegerOverflow=on  InputSameDT=on
  <0 : Outport
  wires:
  Sign1/1 -> Switch1/2, Product1/2, Product5/1
  Product1/1 -> Switch1/1
  Product5/1 -> Switch1/3
  Switch1/1 -> <0/1
  In2/1 -> Sign1/1, Product1/1, Abs/1
  Abs/1 -> Product5/2

== system rov_design_analysis/Thruster  Controller/2. Thruster Allocation- RRC ROV/thruster allocation /Atomic Subsystem4 ==
  In1 : Inport  Port=1  LatchInput=off
  In2 : Inport  Port=2  LatchInput=off
  In3 : Inport  Port=3  LatchInput=off
  Enable : EnablePort
  Subtract : Sum  Inputs=+++  OutScaling=2^-10
  Out1 : Outport
  wires:
  In1/1 -> Subtract/1
  In2/1 -> Subtract/2
  In3/1 -> Subtract/3
  Subtract/1 -> Out1/1

== system rov_design_analysis/Thruster  Controller/2. Thruster Allocation- RRC ROV/thruster allocation /Atomic Subsystem5 ==
  In1 : Inport  Port=1  LatchInput=off
  In2 : Inport  Port=2  LatchInput=off
  In3 : Inport  Port=3  LatchInput=off
  Enable : EnablePort
  Subtract : Sum  Inputs=+++  OutScaling=2^-10
  Out1 : Outport
  wires:
  In1/1 -> Subtract/1
  In2/1 -> Subtract/2
  In3/1 -> Subtract/3
  Subtract/1 -> Out1/1

== system rov_design_analysis/Thruster  Controller/2. Thruster Allocation- RRC ROV/thruster allocation /Atomic Subsystem6 ==
  In1 : Inport  Port=1  LatchInput=off
  In2 : Inport  Port=2  LatchInput=off
  Enable : EnablePort
  Subtract : Sum  OutScaling=2^-10
  Out1 : Outport
  wires:
  In1/1 -> Subtract/1
  In2/1 -> Subtract/2
  Subtract/1 -> Out1/1

== system rov_design_analysis/Thruster  Controller/2. Thruster Allocation- RRC ROV/thruster allocation /Atomic Subsystem7 ==
  1 : Inport  Port=1  LatchInput=off
  2 : Inport  Port=2  LatchInput=off
  Enable : EnablePort
  Subtract : Sum  OutScaling=2^-10
  Out1 : Outport
  wires:
  1/1 -> Subtract/1
  2/1 -> Subtract/2
  Subtract/1 -> Out1/1

== system rov_design_analysis/Thruster  Controller/2. Thruster Allocation- RRC ROV/thruster allocation /Atomic Subsystem8 ==
  In2 : Inport  Port=1  LatchInput=off
  Abs : Abs
  Product1 : Product  OutDataTypeMode=double  SaturateOnIntegerOverflow=on  RndMeth=Zero
  Product5 : Product  OutDataTypeMode=double  SaturateOnIntegerOverflow=on  RndMeth=Zero
  Sign1 : Signum
  Switch1 : Switch  Threshold=1  SaturateOnIntegerOverflow=on  InputSameDT=on
  <0 : Outport
  wires:
  In2/1 -> Sign1/1, Product1/1, Abs/1
  Sign1/1 -> Switch1/2, Product1/2, Product5/1
  Product1/1 -> Switch1/1
  Product5/1 -> Switch1/3
  Switch1/1 -> <0/1
  Abs/1 -> Product5/2

== system rov_design_analysis/Utilities/Euler Transformation 6 DoF/Transformation matrix R/Row1 of T ==
  angular body  velocity : Inport  Port=1  LatchInput=off
  angular position : Inport  Port=2  LatchInput=off
  1 : Fcn  Expr=1
  Dot Product1 : simulink/Math Operations/Dot Product  InputSameDT=on  OutDataType=sfix(16)  OutScaling=2^-10  DoSatur=off
  Mux1 : Mux  Inputs=3
  cX.tY : Fcn  Expr=cos(u[1])*tan(u[2])
  sX.tY : Fcn  Expr=sin(u[1])*tan(u[2])
  angular earth velocity (row 1) : Outport
  wires:
  angular position/1 -> 1/1, sX.tY/1, cX.tY/1
  1/1 -> Mux1/1
  sX.tY/1 -> Mux1/2
  cX.tY/1 -> Mux1/3
  Mux1/1 -> Dot Product1/1
  angular body  velocity/1 -> Dot Product1/2
  Dot Product1/1 -> angular earth velocity (row 1)/1

== system rov_design_analysis/Utilities/Euler Transformation 6 DoF/Transformation matrix R/Row2 of T ==
  "angular body velocity " : Inport  Port=1  LatchInput=off
  angular position : Inport  Port=2  LatchInput=off
  -sX : Fcn  Expr=-sin(u[1])
  0 : Fcn  Expr=0
  Dot Product1 : simulink/Math Operations/Dot Product  InputSameDT=on  OutDataType=sfix(16)  OutScaling=2^-10  DoSatur=off
  Mux1 : Mux  Inputs=3
  cX : Fcn  Expr=cos(u[1])
  angular earth velocity (row 2) : Outport
  wires:
  angular position/1 -> 0/1, cX/1, -sX/1
  0/1 -> Mux1/1
  cX/1 -> Mux1/2
  -sX/1 -> Mux1/3
  Mux1/1 -> Dot Product1/1
  "angular body velocity "/1 -> Dot Product1/2
  Dot Product1/1 -> angular earth velocity (row 2)/1

== system rov_design_analysis/Utilities/Euler Transformation 6 DoF/Transformation matrix R/Row3 of T ==
  "angular body velocity " : Inport  Port=1  LatchInput=off
  angular position : Inport  Port=2  LatchInput=off
  1 : Fcn  Expr=0
  Dot Product1 : simulink/Math Operations/Dot Product  InputSameDT=on  OutDataType=sfix(16)  OutScaling=2^-10  DoSatur=off
  Mux1 : Mux  Inputs=3
  cX/cY : Fcn  Expr=cos(u[1])/cos(u[2])
  sX/cY : Fcn  Expr=sin(u[1])/cos(u[2])
  angular earth velocity (row 3) : Outport
  wires:
  angular position/1 -> 1/1, sX/cY/1, cX/cY/1
  1/1 -> Mux1/1
  sX/cY/1 -> Mux1/2
  cX/cY/1 -> Mux1/3
  Mux1/1 -> Dot Product1/1
  "angular body velocity "/1 -> Dot Product1/2
  Dot Product1/1 -> angular earth velocity (row 3)/1

== system rov_design_analysis/Utilities/Euler Transformation 6 DoF/Transformation matrix T/Row1 of R ==
  translational body velocity : Inport  Port=1  LatchInput=off
  angular position : Inport  Port=2  LatchInput=off
  -sZ.cX+cZ.sY.sX : Fcn  Expr=-sin(u[3])*cos(u[1]) + cos(u[3])*sin(u[2])*sin(u[1])
  Dot Product : simulink/Math Operations/Dot Product  InputSameDT=on  OutDataType=sfix(16)  OutScaling=2^-10  DoSatur=off
  Mux : Mux  Inputs=3
  cY.cZ : Fcn  Expr=cos(u[3]) * cos(u[2])
  sZ.sX+cZ.cX.sY : Fcn  Expr=sin(u[3])*sin(u[1]) + cos(u[3])*cos(u[1])*sin(u[2])
  translational earth velocity (row 1) : Outport
  wires:
  angular position/1 -> cY.cZ/1, -sZ.cX+cZ.sY.sX/1, sZ.sX+cZ.cX.sY/1
  cY.cZ/1 -> Mux/1
  -sZ.cX+cZ.sY.sX/1 -> Mux/2
  sZ.sX+cZ.cX.sY/1 -> Mux/3
  Mux/1 -> Dot Product/1
  translational body velocity/1 -> Dot Product/2
  Dot Product/1 -> translational earth velocity (row 1)/1

== system rov_design_analysis/Utilities/Euler Transformation 6 DoF/Transformation matrix T/Row2 of R ==
  translational body velocity : Inport  Port=1  LatchInput=off
  angular position : Inport  Port=2  LatchInput=off
  -cZ.sX+sY.sZ.cX : Fcn  Expr=-cos(u[3])*sin(u[1]) + sin(u[2])*sin(u[3])*cos(u[1])
  Dot Product1 : simulink/Math Operations/Dot Product  InputSameDT=on  OutDataType=sfix(16)  OutScaling=2^-10  DoSatur=off
  Mux1 : Mux  Inputs=3
  cY.sZ : Fcn  Expr=sin(u[3]) * cos(u[2])
  cZ.cX+sX.sY.sZ : Fcn  Expr=cos(u[3])*cos(u[1]) + sin(u[1])*sin(u[2])*sin(u[3])
  translational earth velocity (row 2) : Outport
  wires:
  angular position/1 -> cY.sZ/1, cZ.cX+sX.sY.sZ/1, -cZ.sX+sY.sZ.cX/1
  cY.sZ/1 -> Mux1/1
  cZ.cX+sX.sY.sZ/1 -> Mux1/2
  -cZ.sX+sY.sZ.cX/1 -> Mux1/3
  Mux1/1 -> Dot Product1/1
  translational body velocity/1 -> Dot Product1/2
  Dot Product1/1 -> translational earth velocity (row 2)/1

== system rov_design_analysis/Utilities/Euler Transformation 6 DoF/Transformation matrix T/Row3 of R ==
  translational body velocity : Inport  Port=1  LatchInput=off
  angular position : Inport  Port=2  LatchInput=off
  -sY : Fcn  Expr=-sin(u[2])
  Dot Product1 : simulink/Math Operations/Dot Product  InputSameDT=on  OutDataType=sfix(16)  OutScaling=2^-10  DoSatur=off
  Mux1 : Mux  Inputs=3
  cY.cX : Fcn  Expr=cos(u[2])*cos(u[1])
  cY.sX : Fcn  Expr=cos(u[2])*sin(u[1])
  translational earth velocity (row 3) : Outport  InitialOutput=0
  wires:
  angular position/1 -> -sY/1, cY.sX/1, cY.cX/1
  -sY/1 -> Mux1/1
  cY.sX/1 -> Mux1/2
  cY.cX/1 -> Mux1/3
  Mux1/1 -> Dot Product1/1
  translational body velocity/1 -> Dot Product1/2
  Dot Product1/1 -> translational earth velocity (row 3)/1

== system rov_design_analysis/Utilities/pipeline  tracking planner  (6 DoF) /coupled input/x25, y=0, z=50 yaw=1.57 ==
  Ground : Ground
  Mux : Mux  Inputs=6
  Start : Constant  Value=10
  Start1 : Constant  Value=15
  Start2 : Constant  Value=0
  3 : Outport
  wires:
  Start1/1 -> Mux/1
  Mux/1 -> 3/1
  Start2/1 -> Mux/6
  Start/1 -> Mux/3
  Ground/1 -> Mux/5, Mux/4, Mux/2

== system rov_design_analysis/Utilities/pipeline  tracking planner  (6 DoF) /coupled input/x=0,y=0, z=0 yaw=0   ==
  Ground : Ground
  Mux : Mux  Inputs=6
  Start : Constant  Value=15
  Start1 : Constant  Value=25
  Start2 : Constant  Value=0
  5 : Outport
  wires:
  Mux/1 -> 5/1
  Start1/1 -> Mux/1
  Start/1 -> Mux/3, Mux/2
  Start2/1 -> Mux/6
  Ground/1 -> Mux/4, Mux/5

== system rov_design_analysis/Utilities/pipeline  tracking planner  (6 DoF) /coupled input/x=0,y=0, z=0 yaw=0  1 ==
  Ground : Ground
  Mux : Mux  Inputs=6
  Start : Constant  Value=15
  Start1 : Constant  Value=25
  Start2 : Constant  Value=1.57
  6 : Outport
  wires:
  Mux/1 -> 6/1
  Start1/1 -> Mux/1
  Start/1 -> Mux/3, Mux/2
  Start2/1 -> Mux/6
  Ground/1 -> Mux/4, Mux/5

== system rov_design_analysis/Utilities/pipeline  tracking planner  (6 DoF) /coupled input/x=0,y=0, z=0 yaw=0  2 ==
  Ground : Ground
  Mux : Mux  Inputs=6
  Start : Constant  Value=15
  Start1 : Constant  Value=25
  Start2 : Constant  Value=0
  0 : Outport
  wires:
  Mux/1 -> 0/1
  Start1/1 -> Mux/1
  Start/1 -> Mux/3, Mux/2
  Start2/1 -> Mux/6
  Ground/1 -> Mux/4, Mux/5

== system rov_design_analysis/Utilities/pipeline  tracking planner  (6 DoF) /coupled input/x=15,y=0, z=45 yaw=0  ==
  Ground : Ground
  Mux : Mux  Inputs=6
  Start1 : Constant  Value=15
  Start2 : Constant  Value=15
  Start3 : Constant  Value=0
  2 : Outport
  wires:
  Mux/1 -> 2/1
  Start1/1 -> Mux/1
  Start2/1 -> Mux/3
  Start3/1 -> Mux/6
  Ground/1 -> Mux/5, Mux/4, Mux/2

== system rov_design_analysis/Utilities/pipeline  tracking planner  (6 DoF) /coupled input/x=25,y=40, z=50 yaw=0 ==
  Ground : Ground
  Mux : Mux  Inputs=6
  Start : Constant  Value=0
  Start1 : Constant  Value=25
  Start2 : Constant  Value=0
  Start3 : Constant  Value=10
  4 : Outport
  wires:
  Start1/1 -> Mux/1
  Mux/1 -> 4/1
  Start/1 -> Mux/6
  Start2/1 -> Mux/2
  Start3/1 -> Mux/3
  Ground/1 -> Mux/4, Mux/5

== system rov_design_analysis/Utilities/pipeline  tracking planner  (6 DoF) /coupled input/x=y=0, z=-50 yaw=0   ==
  Ground : Ground
  Mux : Mux  Inputs=6
  Start : Constant  Value=15
  Start1 : Constant  Value=0
  Start2 : Constant  Value=0
  1 : Outport
  wires:
  Mux/1 -> 1/1
  Start1/1 -> Mux/1
  Start/1 -> Mux/3
  Start2/1 -> Mux/6
  Ground/1 -> Mux/5, Mux/4, Mux/2

== system rov_design_analysis/Utilities/pipeline  tracking planner  (6 DoF) /switching input sequence/decoupled input seq ==
  Demux : Demux  Tag=STV Demux  Outputs=7
  FromWs : FromWorkspace  Tag=STV FromWs  VariableName=tuvar  SampleTime=0  SigBuilderData=DataTag4  VnvData=DataTag5
      SigBuilderData=|
      | channels(1).label = 'Signal 1'
      | channels(1).allXData = {[0 65 65 700]}
      | channels(1).allYData = {[1 1 0 0]}
      | channels(2).label = 'Signal 2'
      | channels(2).allXData = {[0 65 65 150 150 700]}
      | channels(2).allYData = {[0 0 2 2 0 0]}
      | channels(3).label = 'Signal 3'
      | channels(3).allXData = {[0 150 150 230 230 700]}
      | channels(3).allYData = {[0 0 3 3 0 0]}
      | channels(4).label = 'Signal 4'
      | channels(4).allXData = {[0 230 230 290 290 700]}
      | channels(4).allYData = {[0 0 4 4 0 0]}
      | channels(5).label = 'Signal 5'
      | channels(5).allXData = {[0 290 290 350 350 700]}
      | channels(5).allYData = {[0 0 5 5 0 0]}
      | channels(6).label = 'Signal 6'
      | channels(6).allXData = {[0 350 350 400 400 700]}
      | channels(6).allYData = {[0 0 6 6 0 0]}
      | channels(7).label = 'Signal 7'
      | channels(7).allXData = {[0 400 400 689 689 700]}
      | channels(7).allYData = {[0 0 7 7 0 0]}
      | dataSet.timeRange = [0 700]
      | dataSet.name = 'Group 1'
  Signal 1 : Outport  Tag=STV Outport
  Signal 2 : Outport  Tag=STV Outport  Port=2
  Signal 3 : Outport  Tag=STV Outport  Port=3
  Signal 4 : Outport  Tag=STV Outport  Port=4
  Signal 5 : Outport  Tag=STV Outport  Port=5
  Signal 6 : Outport  Tag=STV Outport  Port=6
  Signal 7 : Outport  Tag=STV Outport  Port=7
  wires:
  Demux/1 -> Signal 1/1
  FromWs/1 -> Demux/1
  Demux/2 -> Signal 2/1
  Demux/3 -> Signal 3/1
  Demux/4 -> Signal 4/1
  Demux/5 -> Signal 5/1
  Demux/6 -> Signal 6/1
  Demux/7 -> Signal 7/1

== system rov_design_analysis/ROV Controller /Adaptive PD  Cascaded  Controller - 6 DoF/Body-fixed to Earth_fixed Transformation1/Transformation matrix R/Row1 of T ==
  angular body  velocity : Inport  Port=1  LatchInput=off
  angular position : Inport  Port=2  LatchInput=off
  0 : Fcn  Expr=0
  1 : Fcn  Expr=1
  2 : Fcn  Expr=0
  Dot Product1 : Subsystem  mask(Dot Product){}
      mask help:
      | Inner (dot) product.
      | y=sum(u1.*u2)
      mask init:
      | t=(0:.1:2*pi)';
      | x=cos(t);
      | y=sin(t);
      mask Help: Computes the inner (dot) product of the inputs: sum(u1.*u2).  The inputs are vectors of the same length. Output is a scalar.
      mask Display: plot(0,0,1,1,x*[0.025 0.07]+0.5,y*[0.025 0.07]+0.5)
  Mux1 : Mux  Inputs=3
  angular earth velocity (row 1) : Outport  InitialOutput=0
  wires:
  angular position/1 -> 1/1, 0/1, 2/1
  1/1 -> Mux1/1
  0/1 -> Mux1/2
  2/1 -> Mux1/3
  Mux1/1 -> Dot Product1/1(in_1)
  angular body  velocity/1 -> Dot Product1/2(in_2)
  Dot Product1/1(out_1) -> angular earth velocity (row 1)/1

== system rov_design_analysis/ROV Controller /Adaptive PD  Cascaded  Controller - 6 DoF/Body-fixed to Earth_fixed Transformation1/Transformation matrix R/Row2 of T ==
  "angular body velocity " : Inport  Port=1  LatchInput=off
  angular position : Inport  Port=2  LatchInput=off
  Dot Product1 : Subsystem  mask(Dot Product){}
      mask help:
      | Inner (dot) product.
      | y=sum(u1.*u2)
      mask init:
      | t=(0:.1:2*pi)';
      | x=cos(t);
      | y=sin(t);
      mask Help: Computes the inner (dot) product of the inputs: sum(u1.*u2).  The inputs are vectors of the same length. Output is a scalar.
      mask Display: plot(0,0,1,1,x*[0.025 0.07]+0.5,y*[0.025 0.07]+0.5)
  Mux1 : Mux  Inputs=3
  cX : Fcn  Expr=cos(u[1])
  sX.tY : Fcn  Expr=sin(u[1])*tan(u[2])
  sX/cY : Fcn  Expr=sin(u[1])/cos(u[2])
  angular earth velocity (row 2) : Outport  InitialOutput=0
  wires:
  angular position/1 -> sX.tY/1, cX/1, sX/cY/1
  sX.tY/1 -> Mux1/1
  cX/1 -> Mux1/2
  sX/cY/1 -> Mux1/3
  Mux1/1 -> Dot Product1/1(in_1)
  "angular body velocity "/1 -> Dot Product1/2(in_2)
  Dot Product1/1(out_1) -> angular earth velocity (row 2)/1

== system rov_design_analysis/ROV Controller /Adaptive PD  Cascaded  Controller - 6 DoF/Body-fixed to Earth_fixed Transformation1/Transformation matrix R/Row3 of T ==
  "angular body velocity " : Inport  Port=1  LatchInput=off
  angular position : Inport  Port=2  LatchInput=off
  -sX : Fcn  Expr=-sin(u[1])
  Dot Product1 : Subsystem  mask(Dot Product){}
      mask help:
      | Inner (dot) product.
      | y=sum(u1.*u2)
      mask init:
      | t=(0:.1:2*pi)';
      | x=cos(t);
      | y=sin(t);
      mask Help: Computes the inner (dot) product of the inputs: sum(u1.*u2).  The inputs are vectors of the same length. Output is a scalar.
      mask Display: plot(0,0,1,1,x*[0.025 0.07]+0.5,y*[0.025 0.07]+0.5)
  Mux1 : Mux  Inputs=3
  cX.tY : Fcn  Expr=cos(u[1])*tan(u[2])
  cX/cY : Fcn  Expr=cos(u[1])/cos(u[2])
  angular earth velocity (row 3) : Outport  InitialOutput=0
  wires:
  angular position/1 -> cX.tY/1, -sX/1, cX/cY/1
  cX.tY/1 -> Mux1/1
  -sX/1 -> Mux1/2
  cX/cY/1 -> Mux1/3
  Mux1/1 -> Dot Product1/1(in_1)
  "angular body velocity "/1 -> Dot Product1/2(in_2)
  Dot Product1/1(out_1) -> angular earth velocity (row 3)/1

== system rov_design_analysis/ROV Controller /Adaptive PD  Cascaded  Controller - 6 DoF/Body-fixed to Earth_fixed Transformation1/Transformation matrix T/Row1 of R ==
  translational body velocity : Inport  Port=1  LatchInput=off
  angular position : Inport  Port=2  LatchInput=off
  -sY : Fcn  Expr=-sin(u[2])
  Dot Product : Subsystem  mask(Dot Product){}
      mask help:
      | Inner (dot) product.
      | y=sum(u1.*u2)
      mask init:
      | t=(0:.1:2*pi)';
      | x=cos(t);
      | y=sin(t);
      mask Help: Computes the inner (dot) product of the inputs: sum(u1.*u2).  The inputs are vectors of the same length. Output is a scalar.
      mask Display: plot(0,0,1,1,x*[0.025 0.07]+0.5,y*[0.025 0.07]+0.5)
  Mux : Mux  Inputs=3
  cY.cZ : Fcn  Expr=cos(u[3]) * cos(u[2])
  cY.sZ : Fcn  Expr=sin(u[3]) * cos(u[2])
  translational earth velocity (row 1) : Outport  InitialOutput=0
  wires:
  angular position/1 -> cY.cZ/1, cY.sZ/1, -sY/1
  cY.cZ/1 -> Mux/1
  cY.sZ/1 -> Mux/2
  -sY/1 -> Mux/3
  Mux/1 -> Dot Product/1(in_1)
  translational body velocity/1 -> Dot Product/2(in_2)
  Dot Product/1(out_1) -> translational earth velocity (row 1)/1

== system rov_design_analysis/ROV Controller /Adaptive PD  Cascaded  Controller - 6 DoF/Body-fixed to Earth_fixed Transformation1/Transformation matrix T/Row2 of R ==
  translational body velocity : Inport  Port=1  LatchInput=off
  angular position : Inport  Port=2  LatchInput=off
  -sZ.cX+cZ.sY.sX : Fcn  Expr=-sin(u[3])*cos(u[1]) + cos(u[3])*sin(u[2])*sin(u[1])
  Dot Product1 : Subsystem  mask(Dot Product){}
      mask help:
      | Inner (dot) product.
      | y=sum(u1.*u2)
      mask init:
      | t=(0:.1:2*pi)';
      | x=cos(t);
      | y=sin(t);
      mask Help: Computes the inner (dot) product of the inputs: sum(u1.*u2).  The inputs are vectors of the same length. Output is a scalar.
      mask Display: plot(0,0,1,1,x*[0.025 0.07]+0.5,y*[0.025 0.07]+0.5)
  Mux1 : Mux  Inputs=3
  cY.sX : Fcn  Expr=cos(u[2])*sin(u[1])
  cZ.cX+sX.sY.sZ : Fcn  Expr=cos(u[3])*cos(u[1]) + sin(u[1])*sin(u[2])*sin(u[3])
  translational earth velocity (row 2) : Outport  InitialOutput=0
  wires:
  angular position/1 -> -sZ.cX+cZ.sY.sX/1, cZ.cX+sX.sY.sZ/1, cY.sX/1
  -sZ.cX+cZ.sY.sX/1 -> Mux1/1
  cZ.cX+sX.sY.sZ/1 -> Mux1/2
  cY.sX/1 -> Mux1/3
  Mux1/1 -> Dot Product1/1(in_1)
  translational body velocity/1 -> Dot Product1/2(in_2)
  Dot Product1/1(out_1) -> translational earth velocity (row 2)/1
